simulink library "vmc"  (R2021b)
settings: Solver=VariableStepAuto  StartTime=0.0  StopTime=10.0  RelTol=1e-3
undefined symbols (not defined in the file or in its folder): AVMC_ACCDeltaTqIGain_X_kph, AVMC_ACCDeltaTqIGain_Y_mps2, AVMC_ACCDeltaTqPGain_X_kph, AVMC_ACCDeltaTqPGain_Y_kph, AVMC_ACCLongSteadyCtrl_X_kph, AVMC_AggressJerkPCT4AT_X_kph, AVMC_AggressJerkPCT_X_kph, AVMC_AggressLimitPCT4AT_X_kph, AVMC_AggressLimitPCT_X_kph, AVMC_CCLongSteadyCtrl_X_kph, AVMC_DISCDeltaTqIGain_X_kph, AVMC_DISCDeltaTqIGain_Y_mps2, AVMC_DISCDeltaTqPGain_X_kph, AVMC_DISCDeltaTqPGain_Y_kph, AVMC_DISCTrunAccJerk_X_s, AVMC_DISCTrunAccLimit_X_s, AVMC_ESCRegenOut_X_kph, AVMC_ESCRegenOut_Y_Deg, AVMC_ESCRegenOutEnSpd_X_Deg, AVMC_ISOAccLimit_X_mps, AVMC_ISODecLimit_X_mps, AVMC_ISOJerk_X_mps, AVMC_LatESCRegenOut_X_kph, AVMC_LatESCRegenOut_Y_Deg, AVMC_LongAccDeadZone_X_kph, AVMC_LongAccFiltTsforP2_X_Gps, AVMC_MCPresBaseTq_X_bar, AVMC_MSALongSteadyCtrl_X_kph, AVMC_MSAPedalOvrd2_X_kph, AVMC_MSAPedalOvrd_X_kph, AVMC_MSASpdBand_X_kph, AVMC_MSATqDownEndTq_X_kph, AVMC_MSATqDownTime_X_kph, AVMC_OPDDisSlideRate_X_Deg, AVMC_RDCDetectTime_X_kph, AVMC_RDCDetectTime_Y_pct, AVMC_RDCEnSlideRate_X_Deg, AVMC_RearWhlTqRatio_X_Nm, AVMC_RearWhlTqRatio_Y_gps, AVMC_RearWhlTqSlipGain_X_rat, AVMC_RearWhlTqSlipGain_Y_kph, AVMC_RearWhlTqSTRGGain_X_deg, AVMC_RearWhlTqSTRGGain_Y_kph, AVMC_RWSRrTSA2RWSPos_X_deg, AVMC_RWSSAS2FrtTSA_X_deg, AVMC_RWSVehSPD2RWSCoef_X_kph, AVMC_SoftJerkPCT_X_kph, AVMC_SoftLimitPCT_X_kph, AVMC_StESCYaw_X_kph, AVMC_StESCYaw_Y_Deg, AVMC_StESCYawCom_X_kph, AVMC_StESCYawCom_Y_Gps, AVMC_TMSpdBaseTq_X_rpm, AVMC_VehHoldBDecMap_X_kph, AVMC_VehHoldDecCtrlTime_X_kph, AVMC_VehHoldMCPPass_X_deg, C_TASK_10MS_S, C_TASK_5MS_S, DEG2RAD, ENUM_ACCAVAIL_AVAILABLE ... (+409)
libraries: hcu_lib x74, simulink x68, simulink_extras x3, $bdroot x2
(part 6 of 15)

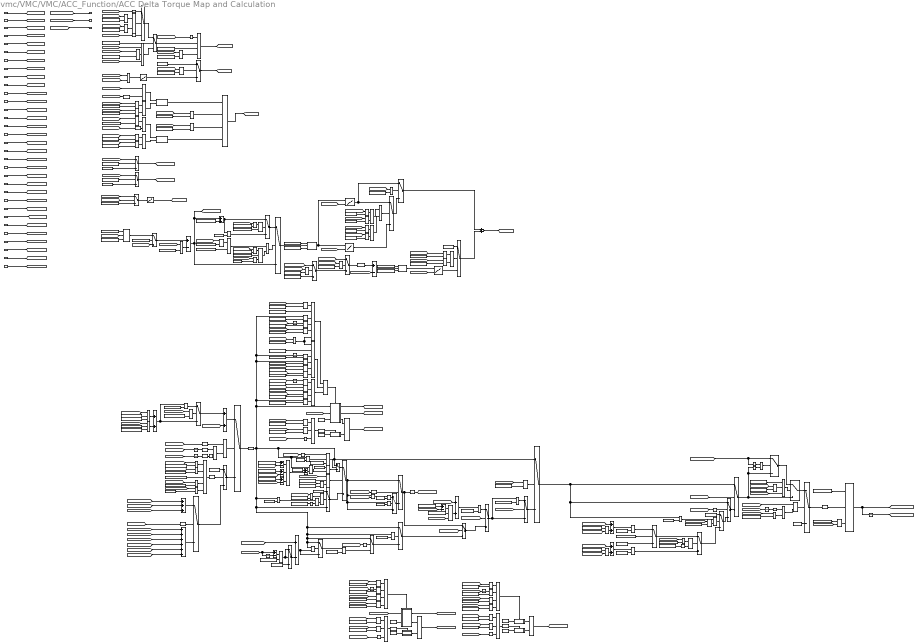
== system vmc/VMC/VMC/ACC_Function/ACC Delta Torque Map and Calculation ==
  note: Deceleration REGEN Torque Control
  note: Deceleration REGEN Torque Control Judgement
  note: Deceleration Torque Control
  note: Deceleration Positive Torque Control
  VVMC_LongAcc_Gps : Inport
  VVMC_ActACCRequiredAccel_mps2 : Inport  Port=2
  VINP_VehSpeed_kph : Inport  Port=3
  VTQD_DriverWhlTqDem_Nm : Inport  Port=4
  VVMC_ADASActive_flg : Inport  Port=5
  VTQD_CoordWhlTqDemFr_Nm : Inport  Port=6
  VTQD_CoordWhlTqDemRr_Nm : Inport  Port=7
  VVMC_ACCPedalOvrd_flg : Inport  Port=8
  VVMC_FeatSetSpdForCalcu_kph : Inport  Port=9
  VVMC_FeatArbitrFinal_enum : Inport  Port=10
  VINP_FrTMSpd_rpm : Inport  Port=11
  VINP_RrTMSpd_rpm : Inport  Port=12
  VINP_MCPressure_bar : Inport  Port=13
  VINP_ESCADASSta_enum : Inport  Port=14
  VINP_FrRBCActive_flg : Inport  Port=15
  VINP_RrRBCActive_flg : Inport  Port=16
  VVMC_FeatReqSpd_kph : Inport  Port=17
  VVMC_MeterIndSpeedForCalcu_kph : Inport  Port=18
  VTQD_SWCResUpSta_flg : Inport  Port=19
  VINP_FrntAxlTrqReqBrk_Nm : Inport  Port=20
  VINP_RearAxlTrqReqBrk_Nm : Inport  Port=21
  VTQR_RrTMTqReq_Nm : Inport  Port=22
  VVMC_ACCVehHoldReq_flg : Inport  Port=23
  VVMC_EstSlope_Deg : Inport  Port=24
  VINP_TargetType_enum : Inport  Port=25
  VVMC_SafetyCtrl_flg : Inport  Port=26
  VTQR_FrTMTqReq_Nm : Inport  Port=27
  task_time_s : Inport  Port=28
  VVMC_TotalAvailBrkRgnTq_Nm : Inport  Port=29
  VVMC_AccelTurnHold_flg : Inport  Port=30
  VVMC_ADASACCSta_enum : Inport  Port=31
  VVMC_TimeGapJudge_flag : Inport  Port=32
  AND{,1,4,10..11,13,15,17..18,20,24,29,31} (13 alike) : Logic  AllPortsSameDT=off  OutDataTypeStr=boolean
  AND12 : Logic  Inputs=3  AllPortsSameDT=off  OutDataTypeStr=boolean
  AND14 : Logic  Operator=OR  AllPortsSameDT=off  OutDataTypeStr=boolean
  AND19 : Logic  Operator=OR  AllPortsSameDT=off  OutDataTypeStr=boolean
  AND2 : Logic  Inputs=4  AllPortsSameDT=off  OutDataTypeStr=boolean
  AND25 : Logic  Inputs=3  AllPortsSameDT=off  OutDataTypeStr=boolean
  AND3 : Logic  Inputs=4  AllPortsSameDT=off  OutDataTypeStr=boolean
  AND30 : Logic  Operator=OR  AllPortsSameDT=off  OutDataTypeStr=boolean
  AND32 : Logic  Inputs=5  AllPortsSameDT=off  OutDataTypeStr=boolean
  AND8 : Logic  Inputs=3  AllPortsSameDT=off  OutDataTypeStr=boolean
  Abs : Abs
  Abs1 : Abs
  Add{,3..4,7..8,10..12,14} (9 alike) : Sum  Inputs=+-
  Add1 : Sum  Inputs=++++++
  Add{5..6,13,15,18,20..21} (7 alike) : Sum
  Add9 : Sum  Inputs=+++
  Cast To Single2 : DataTypeConversion  OutDataTypeStr=single
  Cast To Single3 : DataTypeConversion  OutDataTypeStr=single
  Constant : Constant  Value=TRUE
  Constant1 : Constant  Value=KVMC_ADASNegReqSourceSW_flg
  Constant10 : Constant  Value=KVMC_ADASWhlTqUpperLim_Nm
  Constant100 : Constant  Value=KVMC_ZeroRgnTqSpdCtrlTime_s
  Constant{4,19,22,25,27,29,40,43,45,50..53,58,63..64,66..67,69..70,72..75,81..82,87,89..90,92..93,96,98..99,101,112,114,116..117,119,124..125,129,131..132,149,151,156,163,165,168,170,174} (53 alike) : Constant  Value=ZERO_FLOAT
  Constant11 : Constant  Value=KVMC_ADASWhlTqLowerLim_Nm
  Constant110 : Constant  Value=KVMC_NegReqEnSpd_kph
  Constant113 : Constant  Value=KVMC_ACCLowSpdPosTq_flg
  Constant115 : Constant  Value=KVMC_ACCLowSpdPosTq_flg
  Constant118 : Constant  Value=KVMC_VehHoldTMBaseTqOff_flg
  Constant12 : Constant  Value=KVMC_AccDevLowLim_mps2
  Constant123 : Constant  Value=ENUM_FEATARBITRSTA_DISC
  Constant126 : Constant  Value=KVMC_ReqAccelDeviaEnDec_mps2
  Constant127 : Constant  Value=KVMC_ReqAccelDevia4Tq_flg
  Constant128 : Constant  Value=KVMC_ReqAccelDeviation_mps2
  Constant13 : Constant  Value=KVMC_AccDevUpLim_mps2
  Constant130 : Constant  Value=KVMC_ReqAccelDeviaMinMCP_bar
  Constant138 : Constant  Value=KVMC_ReqAccelLimitSW_flg
  Constant139 : Constant  Value=KVMC_MaxReqAccel_mps2
  Constant14 : Constant  Value=KVMC_ACCSpdDevUpLim_kph
  Constant140 : Constant  Value=KVMC_MinReqAccel_mps2
  Constant146 : Constant  Value=KVMC_ReqAccelDeviaMinMCPSW_flg
  Constant147 : Constant  Value=KVMC_ReqAccelDeviaMinSpd_kph
  Constant148 : Constant  Value=KVMC_ReqAccelDeviaMinSpdSW_flg
  Constant15 : Constant  Value=KVMC_ACCSpdDevLowLim_kph
  Constant157 : Constant  Value=KVMC_AccelTurnHoldZeroTq_flg
  Constant16 : Constant  Value=ENUM_FEATARBITRSTA_ACC
  Constant162 : Constant  Value=KVMC_HoldTqRamp2ZeroSlope_Nmps
  Constant164 : Constant  Value=KVMC_UpHillHoldTqCtrl_flg
  Constant166 : Constant  Value=ENUM_ESCADASSTA_VEHASTANDSTILL
  Constant167 : Constant  Value=KVMC_StandstillTqRamp2ZeroSlope_Nmps
  Constant169 : Constant  Value=KVMC_StandstillTqRampSW_flg
  Constant17 : Constant  Value=ENUM_ADASACCSTA_ACTIVE
  Constant171 : Constant  Value=KVMC_BigDeltaDecGapBand_mps2
  Constant172 : Constant  Value=KVMC_BigDeltaDecJudgeEnBand_mps2
  Constant173 : Constant  Value=KVMC_BigDeltaDecEnGradeBand_deg
  Constant18 : Constant  Value=KVMC_TimeGapTq2Zero_flg
  Constant{2,7..8,20} (4 alike) : Constant  Value=KVMC_HillUpResetTMSpd_rpm
  Constant21 : Constant  Value=ENUM_FEATARBITRSTA_DISC
  Constant23 : Constant  Value=KVMC_ADASNegReqSW_flg
  Constant24 : Constant  Value=KVMC_ACCReqCMdBond_mps2
  Constant26 : Constant  Value=KVMC_AddBRegen2ACCLoop_flg
  Constant3 : Constant  Value=ENUM_ESCADASSTA_VEHASTANDSTILL
  Constant30 : Constant  Value=KVMC_TqSafetyCtrl_flg
  Constant31 : Constant  Value=KVMC_ACCResUpEnAccCMD_mps2
  Constant{6,36..37,62,77,80,88,97} (8 alike) : Constant  Value=KVMC_CutOffNegTqSpd_kph
  Constant38 : Constant  Value=KTQR_FrTMGearEff_c
  Constant39 : Constant  Value=FALSE
  Constant{41,47..48,78..79,91} (6 alike) : Constant  Value=KVMC_ZeroRgnTqSpd_kph
  Constant42 : Constant  Value=KTQD_FrTMTotalGearRatio_gain
  Constant46 : Constant  Value=KVMC_ACCLowSpdTqCtrlSW_flg
  Constant5 : Constant  Value=KVMC_AddBRegen2ACCLoop_flg
  Constant54 : Constant  Value=KVMC_NegReqSwEnSpd_kph
  Constant55 : Constant  Value=KVMC_NegReqSwEnSlope_Deg
  Constant56 : Constant  Value=KVMC_ACCResUpEnGrade_Deg
  Constant57 : Constant  Value=ENUM_TARGETTYPE_NONE
  Constant59 : Constant  Value=KVMC_TqMCPRelFactor_Nm
  Constant60 : Constant  Value=ENUM_FEATARBITRSTA_ACC
  Constant61 : Constant  Value=ENUM_FEATARBITRSTA_ACC
  Constant68 : Constant  Value=KVMC_GradeTqCtrl_flg
  Constant71 : Constant  Value=KVMC_BigDeltaDecGapZeroTq_flg
  Constant76 : Constant  Value=KVMC_DownGradeTqCtrl_flg
  Constant83 : Constant  Value=TRUE
  Constant84 : Constant  Value=KTQD_RrTMTotalGearRatio_gain
  Constant85 : Constant  Value=KTQR_RrTMGearEff_c
  Constant86 : Constant  Value=FALSE
  Constant9 : Constant  Value=KVMC_GravityValue_mps2
  Constant94 : Constant  Value=TRUE
  Constant95 : Constant  Value=FALSE
  Data Type Conversion1 : DataTypeConversion  OutDataTypeStr=single
  Detect Change : simulink/Logic and Bit Operations/Detect Change  vinit=0  OutDataTypeStr=boolean
  Detect Decrease2 : simulink/Logic and Bit Operations/Detect Decrease  vinit=0.0  OutDataTypeStr=boolean
  Detect Decrease3 : simulink/Logic and Bit Operations/Detect Decrease  vinit=0.0  OutDataTypeStr=boolean
  Detect Increase{,1..6,8} (8 alike) : simulink/Logic and Bit Operations/Detect Increase  vinit=0.0  OutDataTypeStr=boolean
  Divide : Product  Inputs=*/*
  Divide1 : Product  Inputs=***
  Divide2 : Product  Inputs=**
  Divide3 : Product  Inputs=*/*
  Divide5 : Product  Inputs=***
  Divide6 : Product  Inputs=**
  Divide7 : Product  Inputs=**
  Equal : RelationalOperator  Operator===  OutDataTypeStr=boolean  RndMeth=Simplest
  Equal1 : RelationalOperator  Operator=<=  OutDataTypeStr=boolean  RndMeth=Simplest
  Equal10 : RelationalOperator  Operator===  OutDataTypeStr=boolean  RndMeth=Simplest
  Equal11 : RelationalOperator  Operator=<  OutDataTypeStr=boolean  RndMeth=Simplest
  Equal12 : RelationalOperator  Operator=>  OutDataTypeStr=boolean  RndMeth=Simplest
  Equal2 : RelationalOperator  Operator=~=  OutDataTypeStr=boolean  RndMeth=Simplest
  Equal3 : RelationalOperator  OutDataTypeStr=boolean  RndMeth=Simplest
  Equal5 : RelationalOperator  OutDataTypeStr=boolean  RndMeth=Simplest
  Equal6 : RelationalOperator  Operator=<  OutDataTypeStr=boolean  RndMeth=Simplest
  Equal7 : RelationalOperator  Operator=>  OutDataTypeStr=boolean  RndMeth=Simplest
  Equal8 : RelationalOperator  Operator=<  OutDataTypeStr=boolean  RndMeth=Simplest
  Equal9 : RelationalOperator  Operator=>  OutDataTypeStr=boolean  RndMeth=Simplest
  InitialCondition: 1 : UnitDelay  SampleTime=-1  HasFrameUpgradeWarning=on
  Logical Operator : Logic  Inputs=4  AllPortsSameDT=off  OutDataTypeStr=boolean
  Logical Operator1 : Logic  Operator=OR  AllPortsSameDT=off  OutDataTypeStr=boolean
  Logical Operator2 : Logic  Inputs=6  AllPortsSameDT=off  OutDataTypeStr=boolean
  Logical Operator3 : Logic  Operator=OR  Inputs=3  AllPortsSameDT=off  OutDataTypeStr=boolean
  Logical Operator4 : Logic  Inputs=6  AllPortsSameDT=off  OutDataTypeStr=boolean
  Logical Operator5 : Logic  Inputs=3  AllPortsSameDT=off  OutDataTypeStr=boolean
  Logical Operator6 : Logic  Inputs=4  AllPortsSameDT=off  OutDataTypeStr=boolean
  Logical Operator7 : Logic  Operator=OR  Inputs=3  AllPortsSameDT=off  OutDataTypeStr=boolean
  Logical Operator8 : Logic  Inputs=4  AllPortsSameDT=off  OutDataTypeStr=boolean
  Logical Operator9 : Logic  Operator=OR  Inputs=3  AllPortsSameDT=off  OutDataTypeStr=boolean
  MVMC_ACCDeltaTqIGain_Z_Nm : Lookup_n-D  BreakpointsForDimension1=AVMC_ACCDeltaTqIGain_Y_mps2  BreakpointsForDimension2=AVMC_ACCDeltaTqIGain_X_kph  Table=MVMC_ACCDeltaTqIGain_Z_Nm  InternalRulePriority=Speed  RndMeth=Simplest  InputSameDT=on
      settings: InputPortMap=u0,u1
  MVMC_ACCDeltaTqPGain_Z_Nm1 : Lookup_n-D  BreakpointsForDimension1=AVMC_ACCDeltaTqPGain_Y_kph  BreakpointsForDimension2=AVMC_ACCDeltaTqPGain_X_kph  Table=MVMC_ACCDeltaTqPGain_Z_Nm  InternalRulePriority=Speed  RndMeth=Simplest  InputSameDT=on
      settings: InputPortMap=u0,u1
  MVMC_DISCDeltaTqIGain_Z_Nm : Lookup_n-D  BreakpointsForDimension1=AVMC_DISCDeltaTqIGain_Y_mps2  BreakpointsForDimension2=AVMC_DISCDeltaTqIGain_X_kph  Table=MVMC_DISCDeltaTqIGain_Z_Nm  InternalRulePriority=Speed  RndMeth=Simplest  InputSameDT=on
      settings: InputPortMap=u0,u1
  MVMC_MCPresBaseTq_Y_Nm : Lookup_n-D  NumberOfTableDimensions=1  BreakpointsForDimension1=AVMC_MCPresBaseTq_X_bar  Table=MVMC_MCPresBaseTq_Y_Nm  InternalRulePriority=Speed  RndMeth=Simplest  InputSameDT=on
  MVMC_TMSpdBaseTq_Y_Nm : Lookup_n-D  NumberOfTableDimensions=1  BreakpointsForDimension1=AVMC_TMSpdBaseTq_X_rpm  Table=MVMC_TMSpdBaseTq_Y_Nm  InternalRulePriority=Speed  RndMeth=Simplest  InputSameDT=on
  Max{,1,4,6..8} (6 alike) : MinMax  Function=max  Inputs=2
  Max2 : MinMax  Inputs=2
  Max3 : MinMax  Inputs=2
  Merge : Merge
  Merge1 : Merge
  Merge2 : Merge
  Min{,1,3..4} (4 alike) : MinMax  Inputs=2
  Min2 : MinMax  Function=max  Inputs=2
  NOT{,1..5,7,9,12..13,20} (11 alike) : Logic  Operator=NOT  AllPortsSameDT=off  OutDataTypeStr=boolean
  OR{,1,6,11,18} (5 alike) : Logic  Operator=OR  AllPortsSameDT=off  OutDataTypeStr=boolean
  OR2 : Logic  Operator=OR  Inputs=3  AllPortsSameDT=off  OutDataTypeStr=boolean
  OR3 : Logic  Operator=OR  Inputs=3  AllPortsSameDT=off  OutDataTypeStr=boolean
  OR5 : Logic  AllPortsSameDT=off  OutDataTypeStr=boolean
  Product1 : Product
  Relational Operator{,2..4,7,16,32..33,38,44,47} (11 alike) : RelationalOperator  Operator=>  OutDataTypeStr=boolean  RndMeth=Simplest
  Relational Operator{1,9,11,14..15,21..23,26,28,30..31,35,41,45,49..50,57,67} (19 alike) : RelationalOperator  Operator=<  OutDataTypeStr=boolean  RndMeth=Simplest
  Relational Operator{8,10,12,24..25,29,36..37,39,42..43} (11 alike) : RelationalOperator  OutDataTypeStr=boolean  RndMeth=Simplest
  Relational Operator{5..6,17,19,55,73} (6 alike) : RelationalOperator  Operator===  OutDataTypeStr=boolean  RndMeth=Simplest
  Relational Operator{18,20,27,34,40,56,66,71,74} (9 alike) : RelationalOperator  Operator=<=  OutDataTypeStr=boolean  RndMeth=Simplest
  Relay : Relay  OnSwitchValue=KVMC_ACCTq2ZeroEnMCPress2_bar  OffSwitchValue=KVMC_ACCTq2ZeroDisMCPress2_bar  OutDataTypeStr=boolean
  Relay1 : Relay  OnSwitchValue=KVMC_ACCTq2ZeroEnMCPress_bar  OffSwitchValue=KVMC_ACCTq2ZeroDisMCPress_bar  OutDataTypeStr=boolean
  SR_Latch : hcu_lib/Basic_Blocks/SR_Latch
  SR_Latch1 : hcu_lib/Basic_Blocks/SR_Latch
  Saturation Dynamic{1,3..5} (4 alike) : simulink/Discontinuities/Saturation Dynamic  OutMin=[]  OutMax=[]  OutDataTypeStr=Inherit: Same as second input  OutDataType=fixdt(1, 16)  OutScaling=2^-10  DoSatur=off
  Switch{,1..19,21..24,27,29,33..35,37..39,41..43} (35 alike) : Switch  Criteria=u2 > Threshold
  Triggered Subsystem : Subsystem  TreatAsAtomicUnit=on
  Triggered Subsystem1 : Subsystem  TreatAsAtomicUnit=on
  Triggered Subsystem2 : Subsystem  TreatAsAtomicUnit=on
  Triggered Subsystem3 : Subsystem  TreatAsAtomicUnit=on
  Triggered Subsystem4 : Subsystem  TreatAsAtomicUnit=on
  Triggered Subsystem5 : Subsystem  TreatAsAtomicUnit=on
  Unit Delay{,1..9} (10 alike) : UnitDelay  SampleTime=-1  HasFrameUpgradeWarning=on
  u2 > 0 : Switch  Criteria=u2 > Threshold
  u2 > 0 (1) : Switch  Criteria=u2 > Threshold
  u2 > 0 (3) : Switch  Criteria=u2 > Threshold
  u2 > 0 (4) : Switch  Criteria=u2 > Threshold
  VVMC_ADASWhlTqCal_Nm : Outport
  VVMC_ADASNegReq_flg : Outport  Port=2
  VVMC_ACCLowSpdTqCtrl_flg : Outport  Port=3
  wires:
  VVMC_FeatReqSpd_kph/1 -> [VVMC_FeatReqSpd_kph]
  [VINP_RrTMSpd_rpm] -> Relational Operator2/1
  [VVMC_ACCVehHoldReq_flg] -> AND4/1
  MVMC_MCPresBaseTq_Y_Nm/1 -> [VVMC_MCPresBaseTq_Nm]  "VVMC_MCPresBaseTq_Nm"
  Switch1/1 -> MVMC_MCPresBaseTq_Y_Nm/1
  [VINP_MCPressure_bar] -> Switch1/1
  Relational Operator/1 -> OR/1
  Equal/1 -> AND1/1
  OR/1 -> SR_Latch/2
  [VINP_FrTMSpd_rpm] -> Relational Operator/1
  [VINP_ESCADASSta_enum] -> Equal/1
  [VINP_RrTMSpd_rpm] -> Relational Operator4/1
  AND1/1 -> SR_Latch1/1
  Relational Operator2/1 -> OR/2
  OR1/1 -> SR_Latch1/2
  Constant19/1 -> Switch1/3
  Constant8/1 -> Relational Operator3/2
  Relational Operator4/1 -> OR1/2
  [VVMC_MCPreBaseTqEn_flg] -> Switch1/2
  [VINP_FrTMSpd_rpm] -> Relational Operator3/1
  Constant7/1 -> Relational Operator4/2
  Constant2/1 -> Relational Operator2/2
  Detect Increase3/1 -> AND1/2
  SR_Latch/1 -> AND3/1  "VVMC_HillUpHoldReqEn_flg"
  AND3/1 -> [VVMC_MCPreBaseTqEn_flg]  "VVMC_MCPreBaseTqEn_flg"
  SR_Latch1/1 -> AND3/4  "VVMC_HillUpESCStaEn_flg"
  Constant3/1 -> Equal/2
  Constant20/1 -> Relational Operator/2
  Relational Operator3/1 -> OR1/1
  VINP_FrTMSpd_rpm/1 -> [VINP_FrTMSpd_rpm]
  VINP_RrTMSpd_rpm/1 -> [VINP_RrTMSpd_rpm]
  VINP_MCPressure_bar/1 -> [VINP_MCPressure_bar]
  VINP_ESCADASSta_enum/1 -> [VINP_ESCADASSta_enum]
  VINP_FrRBCActive_flg/1 -> [VINP_FrRBCActive_flg]
  VINP_RrRBCActive_flg/1 -> [VINP_RrRBCActive_flg]
  VVMC_FeatArbitrFinal_enum/1 -> [VVMC_FeatArbitrFinal_enum]
  VVMC_LongAcc_Gps/1 -> [VVMC_LongAcc_Gps]
  VVMC_ActACCRequiredAccel_mps2/1 -> [VVMC_ActACCRequiredAccel_mps2]
  VINP_VehSpeed_kph/1 -> [VINP_VehSpeed_kph]
  VTQD_DriverWhlTqDem_Nm/1 -> [VTQD_DriverWhlTqDem_Nm]
  VVMC_ADASActive_flg/1 -> [VVMC_ADASActive_flg]
  [VVMC_ADASWhlTqCal_Nm] -> VVMC_ADASWhlTqCal_Nm/1
  VTQD_CoordWhlTqDemFr_Nm/1 -> [VTQD_CoordWhlTqDemFr_Nm]
  VTQD_CoordWhlTqDemRr_Nm/1 -> [VTQD_CoordWhlTqDemRr_Nm]
  VVMC_ACCPedalOvrd_flg/1 -> [VVMC_ACCPedalOvrd_flg]
  VVMC_FeatSetSpdForCalcu_kph/1 -> [VVMC_FeatSetSpdForCalcu_kph]
  VINP_RearAxlTrqReqBrk_Nm/1 -> [VINP_RearAxlTrqReqBrk_Nm]
  VINP_FrntAxlTrqReqBrk_Nm/1 -> [VINP_FrntAxlTrqReqBrk_Nm]
  VTQD_SWCResUpSta_flg/1 -> [VTQD_SWCResUpSta_flg]
  VVMC_MeterIndSpeedForCalcu_kph/1 -> [VVMC_MeterIndSpeedForCalcu_kph]
  [VTQD_SWCResUpSta_flg] -> Detect Increase2/1
  AND4/1 -> SR_Latch/1
  [VVMC_ActACCRequiredAccel_mps2] -> Relational Operator7/1
  Constant31/1 -> Relational Operator7/2
  [VTQD_SWCResUpSta_flg] -> Detect Increase3/1
  [VINP_FrntAxlTrqReqBrk_Nm] -> Switch3/1
  [VINP_RearAxlTrqReqBrk_Nm] -> Switch4/1
  Constant25/1 -> Switch3/3
  Constant27/1 -> Switch4/3
  Constant26/1 -> Switch4/2
  Switch4/1 -> [VVMC_RearAxlTrqReqBrk_Nm]  "VVMC_RearAxlTrqReqBrk_Nm"
  Switch3/1 -> [VVMC_FrntAxlTrqReqBrk_Nm]  "VVMC_FrntAxlTrqReqBrk_Nm"
  Constant5/1 -> Switch3/2
  [VVMC_ADASNegReq_flg] -> VVMC_ADASNegReq_flg/1
  VTQR_RrTMTqReq_Nm/1 -> [VTQR_RrTMTqReq_Nm]
  VVMC_ACCVehHoldReq_flg/1 -> [VVMC_ACCVehHoldReq_flg]
  [VVMC_EstSlope_Deg] -> Relational Operator16/1
  Relational Operator16/1 -> AND3/3
  Constant56/1 -> Relational Operator16/2
  VVMC_EstSlope_Deg/1 -> [VVMC_EstSlope_Deg]
  VINP_TargetType_enum/1 -> [VINP_TargetType_enum]
  VVMC_SafetyCtrl_flg/1 -> [VVMC_SafetyCtrl_flg]
  VTQR_FrTMTqReq_Nm/1 -> [VTQR_FrTMTqReq_Nm]
  [VVMC_ACCLowSpdTqCtrl_flg] -> VVMC_ACCLowSpdTqCtrl_flg/1
  task_time_s/1 -> [task_time_s]
  MVMC_TMSpdBaseTq_Y_Nm/1 -> Switch/3
  [VVMC_ActACCRequiredAccel_mps2] -> Relational Operator1/1
  AND15/1 -> Switch/2
  Relay/1 -> Switch13/1
  Constant24/1 -> Relational Operator1/2
  [VVMC_ACCVehHoldReq_flg] -> AND15/1
  Switch2/1 -> AND2/2  "VVMC_ADASNegReqAct_flg"
  AND2/1 -> [VVMC_ADASNegReq_flg]  "VVMC_ADASNegReq_flg"
  [VINP_FrRBCActive_flg] -> OR2/1
  Constant23/1 -> AND2/3
  Constant1/1 -> Switch2/2
  [VINP_RrTMSpd_rpm] -> Min/2
  [VVMC_MCPreBaseTqEn_flg] -> NOT2/1
  Equal5/1 -> AND2/4
  [VINP_VehSpeed_kph] -> Equal5/1
  [VINP_FrTMSpd_rpm] -> Min/1
  Switch13/1 -> Switch2/1
  Constant110/1 -> Equal5/2
  [VINP_MCPressure_bar] -> Relay/1
  [VINP_VehSpeed_kph] -> Equal1/1
  Equal3/1 -> AND10/2
  Relay1/1 -> Switch13/3
  Relational Operator1/1 -> OR2/2
  Switch/1 -> [VVMC_TMSpdBaseTq_Nm]  "VVMC_TMSpdBaseTq_Nm"
  Constant54/1 -> Equal1/2
  Constant118/1 -> AND15/2
  [VINP_MCPressure_bar] -> Relay1/1
  AND10/1 -> Switch13/2
  Constant55/1 -> Equal3/2
  [VVMC_EstSlope_Deg] -> Equal3/1
  Equal1/1 -> AND10/1
  Min/1 -> MVMC_TMSpdBaseTq_Y_Nm/1
  NOT2/1 -> AND2/1
  OR2/1 -> Switch2/3
  [VINP_RrRBCActive_flg] -> OR2/3
  Constant119/1 -> Switch/1
  Switch29/1 -> Switch22/3
  [VINP_VehSpeed_kph] -> Relational Operator21/1
  [VINP_VehSpeed_kph] -> Relational Operator20/1
  Relational Operator11/1 -> Logical Operator/2
  Merge2/1 -> [VVMC_ZeroRgnTqSpdCtrl_flg]  "VVMC_ZeroRgnTqSpdCtrl_flg"
  [VVMC_ActACCRequiredAccel_mps2] -> Relational Operator37/1
  Relational Operator50/1 -> Switch29/2
  Constant48/1 -> Add4/1
  Relational Operator73/1 -> OR6/2
  Constant86/1 -> Triggered Subsystem3/1(In1)
  Relational Operator31/1 -> Logical Operator4/1
  Relational Operator39/1 -> Logical Operator6/1
  [VVMC_ActACCRequiredAccel_mps2] -> Relational Operator41/1
  NOT12/1 -> AND14/2
  Logical Operator2/1 -> OR3/2
  Constant93/1 -> Relational Operator42/2
  Relational Operator25/1 -> Logical Operator2/3
  Max1/1 -> Switch23/1
  Detect Increase5/1 -> Triggered Subsystem3/Trigger
  Constant115/1 -> NOT12/1
  Unit Delay4/1 -> NOT4/1
  Logical Operator/1 -> OR3/3
  Detect Increase6/1 -> Triggered Subsystem5/Trigger
  [VVMC_LastADASWhlTqCal_Nm] -> Add12/1
  [VINP_VehSpeed_kph] -> Relational Operator8/1
  Switch8/1 -> Switch43/3
  [VVMC_ADASActive_flg] -> NOT1/1
  Constant63/1 -> Min2/2
  Logical Operator3/1 -> Detect Increase/1
  Constant29/1 -> Relational Operator10/2
  Triggered Subsystem2/1(Out1) -> Merge/2
  Relational Operator8/1 -> Logical Operator3/1
  Unit Delay/1 -> Relational Operator12/1
  [VVMC_TMSpdBaseTq_Nm] -> Add1/3
  Logical Operator1/1 -> Switch6/2
  Constant36/1 -> Relational Operator11/2
  NOT1/1 -> Logical Operator3/3
  [VINP_MCPressure_bar] -> Add11/1, Unit Delay5/1
  [VVMC_FrntAxlTrqReqBrk_Nm] -> Add1/5
  [VTQD_CoordWhlTqDemFr_Nm] -> Add9/1
  Divide2/1 -> Switch15/1, Switch15/2
  Constant92/1 -> Relational Operator41/2
  Constant74/1 -> Switch5/3
  Constant84/1 -> Divide5/2
  Relational Operator15/1 -> Logical Operator/4
  Constant11/1 -> Max6/1
  Constant113/1 -> AND8/3
  [VVMC_ActACCRequiredAccel_mps2] -> Relational Operator10/1
  Triggered Subsystem3/1(Out1) -> Merge1/2
  Constant114/1 -> Relational Operator49/2
  AND13/1 -> Switch21/2
  Constant69/1 -> Switch15/3
  [VVMC_LastADASWhlTqCal_Nm] -> Relational Operator39/1
  Add14/1 -> Divide3/1
  Constant101/1 -> Max2/2
  Switch23/1 -> Switch17/3
  Constant70/1 -> Relational Operator26/2
  [VVMC_ADASActive_flg] -> OR5/1
  Abs1/1 -> Relational Operator18/2
  [VVMC_MCPresBaseTq_Nm] -> Add1/4
  [VINP_VehSpeed_kph] -> Relational Operator44/1
  Switch11/1 -> u2 > 0 (3)/3, u2 > 0 (4)/3, Abs1/1
  Constant61/1 -> Relational Operator19/2
  Abs/1 -> Relational Operator18/1
  Relational Operator19/1 -> AND12/2
  Constant87/1 -> Relational Operator37/2
  Constant68/1 -> Logical Operator2/2
  Switch10/1 -> Min2/1
  Constant64/1 -> Relational Operator22/2
  Constant10/1 -> Saturation Dynamic3/1
  Min2/1 -> Switch16/3
  [VTQR_RrTMTqReq_Nm] -> Divide5/1
  Triggered Subsystem1/2(Out2) -> [VVMC_ACCLowSpdCtrlEnSpd_kph]  "VVMC_ACCLowSpdCtrlEnSpd_kph"
  NOT9/1 -> Logical Operator9/3
  Switch6/1 -> Cast To Single2/1
  Logical Operator8/1 -> Triggered Subsystem4/Trigger
  Cast To Single2/1 -> Relational Operator9/1, Switch10/1, Switch16/1, Relational Operator26/1, Switch19/1, Switch21/3, Relational Operator49/1, Switch17/1, Switch27/1, Max4/1, Relational Operator47/1, Relational Operator30/1, Unit Delay3/1, Relational Operator23/1, Relational Operator15/1, Triggered Subsystem1/1(In1)  "VVMC_OriADASWhlTq_Nm"
  Add11/1 -> Divide2/1
  Unit Delay7/1 -> [VVMC_LastACCLowSpdTq_Nm]
  Detect Increase1/1 -> Logical Operator1/1
  [VVMC_ZeroRgnTqSpdCtrl_flg] -> Switch24/2
  Triggered Subsystem/1(Out1) -> Merge1/1
  Add15/1 -> Max2/1
  Constant46/1 -> Logical Operator5/2
  Add5/1 -> Switch6/1
  Relational Operator34/1 -> Logical Operator6/4
  Divide1/1 -> Add13/1
  Triggered Subsystem4/1(Out1) -> [VVMC_ZeroRgnTqSpdCtrlTq_Nm]  "VVMC_ZeroRgnTqSpdCtrlTq_Nm"
  Unit Delay9/1 -> Relational Operator42/1
  Detect Decrease2/1 -> Switch8/2
  Add13/1 -> Switch9/3, Min3/1
  [VVMC_SafetyCtrl_flg] -> AND12/3
  [VVMC_LastADASWhlTqCal_Nm] -> Relational Operator45/1
  Relational Operator32/1 -> Logical Operator4/6, Logical Operator2/1
  [VVMC_LastADASWhlTqCal_Nm] -> Triggered Subsystem4/1(In1)
  Constant96/1 -> Relational Operator43/2
  [VINP_VehSpeed_kph] -> Relational Operator40/1
  Constant94/1 -> Triggered Subsystem4/2(In2)
  Divide/1 -> Add/2
  Constant67/1 -> Relational Operator25/2
  Constant90/1 -> Relational Operator39/2
  Relational Operator44/1 -> Logical Operator9/1
  Relational Operator30/1 -> Logical Operator4/3
  Switch21/1 -> Switch12/3
  [VVMC_ActACCRequiredAccel_mps2] -> Unit Delay6/1
  [VVMC_ActACCRequiredAccel_mps2] -> Relational Operator43/1
  Constant97/1 -> Relational Operator44/2
  [VVMC_ADASActive_flg] -> NOT9/1
  Add/1 -> Max4/2
  Relational Operator29/1 -> Logical Operator4/4
  Relational Operator45/1 -> Logical Operator8/1
  Constant80/1 -> Relational Operator34/2
  Constant81/1 -> Relational Operator35/2
  Triggered Subsystem5/1(Out1) -> Merge2/2
  Constant98/1 -> Relational Operator45/2
  Constant95/1 -> Triggered Subsystem5/1(In1)
  Constant6/1 -> Relational Operator8/2
  [VVMC_ActACCRequiredAccel_mps2] -> Unit Delay9/1
  Switch18/1 -> Switch24/3
  Add1/1 -> Switch8/3
  Constant100/1 -> Divide3/2
  Triggered Subsystem4/2(Out2) -> Merge2/1
  Constant89/1 -> Max1/2
  Switch7/1 -> Switch11/3
  [VVMC_FeatArbitrFinal_enum] -> Relational Operator19/1
  [VVMC_RgnProhibited_flg] -> Switch23/2
  [VINP_VehSpeed_kph] -> Relational Operator31/1
  [task_time_s] -> Divide3/3
  Merge1/1 -> [VVMC_RgnProhibited_flg]  "VVMC_RgnProhibited_flg"
  Constant53/1 -> Switch21/1
  Relational Operator38/1 -> Logical Operator7/1
  [VVMC_LastADASWhlTqCal_Nm] -> Abs/1, u2 > 0 (4)/1
  Constant88/1 -> Relational Operator38/2
  Triggered Subsystem1/3(Out3) -> Merge/1
  [VVMC_ADASActive_flg] -> NOT7/1
  Relational Operator36/1 -> Logical Operator6/2
  Logical Operator6/1 -> Triggered Subsystem/Trigger
  Max2/1 -> Switch24/1
  Constant82/1 -> Relational Operator36/2
  Constant99/1 -> Add14/1
  [VINP_VehSpeed_kph] -> Relational Operator34/1
  Unit Delay8/1 -> Relational Operator36/1
  Relational Operator35/1 -> Logical Operator6/3
  NOT7/1 -> Logical Operator7/3
  Relational Operator12/1 -> Logical Operator/1
  [VVMC_LastACCLowSpdTq_Nm] -> Max/2
  Switch12/1 -> Switch29/3, Relational Operator50/1, Max/1, Switch22/1
  Switch15/1 -> Add12/2
  Constant117/1 -> Max3/2
  Add9/1 -> Switch8/1
  [VVMC_ActACCRequiredAccel_mps2] -> Relational Operator24/1
  [VVMC_ACCLowSpdCtrlEnSpd_kph] -> Add4/2
  [VVMC_ActACCRequiredAccel_mps2] -> Relational Operator35/1
  Min1/1 -> Switch27/3
  Detect Increase/1 -> Triggered Subsystem2/Trigger
  Relational Operator20/1 -> AND13/1
  Relational Operator47/1 -> AND8/2
  Max/1 -> Max3/1
  Relational Operator43/1 -> Logical Operator9/2
  Constant47/1 -> Add3/1
  Logical Operator9/1 -> Detect Increase6/1
  [VVMC_ACCLowSpdTqCtrl_flg] -> Detect Increase4/1
  Constant4/1 -> Relational Operator24/2
  Unit Delay5/1 -> Add11/2
  Max3/1 -> Switch29/1
  Detect Increase4/1 -> Switch22/2
  Constant78/1 -> Relational Operator32/2
  Constant79/1 -> Relational Operator33/2
  [VINP_VehSpeed_kph] -> Relational Operator32/1
  [VVMC_ACCLowSpdCtrlEnSpd_kph] -> Relational Operator33/1
  Constant76/1 -> Logical Operator4/2
  [VVMC_ZeroRgnTqSpdCtrlTq_Nm] -> Add14/2
  Constant77/1 -> Relational Operator31/2
  Constant75/1 -> Relational Operator30/2
  Logical Operator4/1 -> OR3/1
  Constant73/1 -> Relational Operator29/2
  Relational Operator42/1 -> Logical Operator8/2
  Constant72/1 -> Relational Operator28/2
  [VVMC_ADASActive_flg] -> Detect Increase1/1
  Relational Operator28/1 -> Logical Operator4/5
  AND12/1 -> u2 > 0 (3)/2
  [VVMC_ActACCRequiredAccel_mps2] -> Relational Operator28/1
  [VVMC_RearAxlTrqReqBrk_Nm] -> Add1/6
  Constant40/1 -> Relational Operator14/2
  Relational Operator41/1 -> Logical Operator8/3
  Constant83/1 -> Triggered Subsystem/1(In1)
  Switch24/1 -> Switch23/3, Max1/1
  OR6/1 -> OR5/2
  [VINP_VehSpeed_kph] -> Unit Delay/1
  [VINP_VehSpeed_kph] -> Triggered Subsystem1/2(In2)
  Unit Delay3/1 -> Relational Operator25/1
  Relational Operator26/1 -> Switch19/2
  AND14/1 -> AND13/2
  Logical Operator7/1 -> Detect Increase5/1
  OR5/1 -> Switch5/2
  Constant38/1 -> Divide1/3
  Switch22/1 -> Unit Delay7/1, Switch18/1  "VVMC_ACCLowSpdTq_Nm"
  [VVMC_ACCLowSpdTqCtrl_flg] -> Logical Operator5/1
  Saturation Dynamic3/1 -> [VVMC_ADASWhlTqCal_Nm], InitialCondition: 1/1  "VVMC_ADASWhlTqCal_Nm"
  OR3/1 -> Triggered Subsystem1/Trigger
  Relational Operator23/1 -> Logical Operator2/4
  [VVMC_ActACCRequiredAccel_mps2] -> Relational Operator22/1
  [VTQR_FrTMTqReq_Nm] -> Divide1/1
  Switch27/1 -> Switch12/1
  u2 > 0 (4)/1 -> u2 > 0 (3)/1
  Relational Operator21/1 -> Logical Operator2/5
  Constant62/1 -> Relational Operator21/2
  Max6/1 -> Saturation Dynamic3/3
  Relational Operator10/1 -> Logical Operator3/2
  Unit Delay6/1 -> Relational Operator29/1
  Relational Operator18/1 -> u2 > 0 (4)/2
  [VINP_VehSpeed_kph] -> Relational Operator11/1
  Constant/1 -> Triggered Subsystem1/3(In3)
  Add10/1 -> Divide/3
  Constant112/1 -> Relational Operator47/2
  [VVMC_MCPreBaseTqEn_flg] -> Switch11/2
  Logical Operator5/1 -> Switch12/2
  AND/1 -> Logical Operator1/2
  Constant52/1 -> Min1/1
  [VVMC_ACCVehHoldReq_flg] -> NOT3/1
  Relational Operator9/1 -> Switch10/2
  Add12/1 -> Relational Operator9/2, Switch10/3  "VVMC_ACCTqRampOutByMCP_Nm"
  Add4/1 -> Divide/2
  [VVMC_LastADASWhlTqCal_Nm] -> Add15/1
  Add3/1 -> Divide/1
  [VVMC_ADASNegReq_flg] -> Detect Decrease2/1
  Divide5/1 -> Add13/2
  Relational Operator24/1 -> Switch17/2
  Constant85/1 -> Divide5/3
  Constant50/1 -> Add10/1
  Relational Operator37/1 -> Logical Operator7/2
  Constant37/1 -> Relational Operator12/2
  [VVMC_ACCDeltaTq_Nm] -> Add9/3
  Relational Operator22/1 -> Logical Operator2/6
  Constant66/1 -> Relational Operator23/2
  Constant45/1 -> Relational Operator15/2
  Relational Operator40/1 -> Logical Operator8/4
  InitialCondition: 1/1 -> [VVMC_LastADASWhlTqCal_Nm]  "VVMC_LastADASWhlTqCal_Nm"
  Constant42/1 -> Divide1/2
  [VVMC_ActACCRequiredAccel_mps2] -> Relational Operator14/1
  Relational Operator14/1 -> Logical Operator/3
  [VVMC_ACCDeltaTq_Nm] -> Add1/2
  u2 > 0 (3)/1 -> Switch5/1
  [VVMC_LastADASWhlTqCal_Nm] -> Add1/1
  [VVMC_ACCLowSpdTqLimit_Nm] -> Add10/2
  Triggered Subsystem1/1(Out1) -> [VVMC_ACCLowSpdTqLimit_Nm]  "VVMC_ACCLowSpdTqLimit_Nm"
  NOT3/1 -> Switch7/2
  Constant116/1 -> Relational Operator50/2
  Relational Operator33/1 -> Logical Operator5/3
  [VINP_VehSpeed_kph] -> Add3/2
  Constant51/1 -> Add/1
  [VVMC_ACCLowSpdTqCtrl_flg] -> Switch18/2
  [VTQD_CoordWhlTqDemRr_Nm] -> Add9/2
  Merge/1 -> [VVMC_ACCLowSpdTqCtrl_flg]  "VVMC_ACCLowSpdTqCtrl_flg"
  [VVMC_ACCPedalOvrd_flg] -> Unit Delay4/1
  Constant39/1 -> Triggered Subsystem2/1(In1)
  Constant91/1 -> Relational Operator40/2
  Constant41/1 -> Relational Operator20/2
  Divide3/1 -> Add15/2
  [VVMC_ACCDeltaTq_Nm] -> Add5/2
  [VINP_VehSpeed_kph] -> Relational Operator38/1
  Cast To Single3/1 -> Saturation Dynamic3/2
  Constant59/1 -> Divide2/2
  Switch5/1 -> Cast To Single3/1
  Relational Operator49/1 -> AND14/1
  AND8/1 -> Switch27/2
  Constant30/1 -> AND12/1
  [VVMC_ActACCRequiredAccel_mps2] -> Unit Delay8/1
  Switch17/1 -> Relational Operator71/1, Switch7/1, Switch11/1
  NOT13/1 -> AND8/1
  [VVMC_ADASNegReq_flg] -> NOT13/1
  Constant12/1 -> Saturation Dynamic4/3
  Saturation Dynamic4/1 -> MVMC_DISCDeltaTqIGain_Z_Nm/1, MVMC_ACCDeltaTqIGain_Z_Nm/1  "VVMC_ActAccDev_mps2"
  Switch33/1 -> Add6/1  "VVMC_ACCDeltaTqIGain_Nm"
  Saturation Dynamic5/1 -> MVMC_ACCDeltaTqPGain_Z_Nm1/1  "VVMC_ACCActSpdDev_kph"
  [VVMC_LongAcc_Gps] -> Product1/1
  Constant16/1 -> Relational Operator5/2
  [VVMC_FeatArbitrFinal_enum] -> Relational Operator6/1
  [VVMC_FeatArbitrFinal_enum] -> Relational Operator5/1
  [VVMC_FeatReqSpd_kph] -> u2 > 0 (1)/1
  Constant15/1 -> Saturation Dynamic5/3
  Equal2/1 -> AND11/1
  Constant128/1 -> Add18/2
  Product1/1 -> Add7/2
  Constant21/1 -> Relational Operator6/2
  Constant60/1 -> Relational Operator17/2
  u2 > 0/1 -> Data Type Conversion1/1
  u2 > 0 (1)/1 -> u2 > 0/3
  [VVMC_MeterIndSpeedForCalcu_kph] -> Add8/2
  Add7/1 -> [VVMC_ACCDeltaAccel_mps2], Add18/1, Switch35/3
  Switch38/1 -> Switch35/1
  Constant127/1 -> AND18/2
  [VVMC_LongAcc_Gps] -> Equal6/1
  AND17/1 -> AND19/1
  [VVMC_ActACCRequiredAccel_mps2] -> Equal7/1
  [VINP_VehSpeed_kph] -> MVMC_DISCDeltaTqIGain_Z_Nm/2
  Relational Operator56/1 -> AND18/1
  Constant125/1 -> Equal7/2
  [VINP_TargetType_enum] -> Equal2/1
  MVMC_DISCDeltaTqIGain_Z_Nm/1 -> Switch33/1, Switch34/1  "VVMC_DISCDeltaTqIGain_Nm"
  Constant124/1 -> Equal6/2
  Data Type Conversion1/1 -> Add8/1
  Relational Operator5/1 -> u2 > 0/2
  Add6/1 -> [VVMC_ACCDeltaTq_Nm]  "VVMC_ACCDeltaTq_Nm"
  MVMC_ACCDeltaTqIGain_Z_Nm/1 -> Switch34/3  "VVMC_ACCDeltaTqIGain_Nm"
  Add18/1 -> Min4/1, Switch38/1
  Constant13/1 -> Saturation Dynamic4/1
  [VVMC_FeatArbitrFinal_enum] -> Relational Operator55/1
  Relational Operator55/1 -> Switch33/2
  Constant9/1 -> Product1/2
  [VINP_VehSpeed_kph] -> MVMC_ACCDeltaTqIGain_Z_Nm/2
  Equal6/1 -> AND17/1
  Add8/1 -> Saturation Dynamic5/2
  [VINP_VehSpeed_kph] -> MVMC_ACCDeltaTqPGain_Z_Nm1/2
  Constant129/1 -> Min4/2
  Switch35/1 -> Saturation Dynamic4/2
  Constant123/1 -> Relational Operator55/2
  Constant22/1 -> u2 > 0 (1)/3
  Constant14/1 -> Saturation Dynamic5/1
  Equal7/1 -> AND17/2
  AND11/1 -> Switch14/2
  Relational Operator6/1 -> u2 > 0 (1)/2
  [VVMC_FeatSetSpdForCalcu_kph] -> u2 > 0/1
  MVMC_ACCDeltaTqPGain_Z_Nm1/1 -> Switch14/3
  AND18/1 -> OR11/1
  Relational Operator17/1 -> AND11/2
  [VVMC_FeatArbitrFinal_enum] -> Relational Operator17/1
  Constant57/1 -> Equal2/2
  Switch34/1 -> Switch33/3
  Constant58/1 -> Switch14/1
  Switch14/1 -> Add6/2  "VVMC_ACCDeltaTqPGain_Nm"
  AND19/1 -> Switch34/2
  Constant131/1 -> Equal8/2
  [VVMC_ActACCRequiredAccel_mps2] -> Equal8/1
  Equal8/1 -> AND20/1
  AND20/1 -> AND19/2
  Equal9/1 -> AND20/2
  [VVMC_ACCDeltaAccel_mps2] -> Equal9/1
  Constant132/1 -> Equal9/2
  Constant126/1 -> Relational Operator56/2
  [VVMC_ActACCRequiredAccel_mps2] -> Relational Operator56/1
  Max4/1 -> Min1/2
  Switch19/1 -> Switch18/3
  [VINP_MCPressure_bar] -> Relational Operator57/1
  Constant130/1 -> Relational Operator57/2
  Relational Operator57/1 -> AND24/1
  Min4/1 -> Switch38/3
  AND24/1 -> Switch38/2
  Constant146/1 -> AND24/2
  OR11/1 -> Switch35/2
  Constant148/1 -> AND25/2
  Constant147/1 -> Relational Operator66/2
  [VINP_VehSpeed_kph] -> Relational Operator66/1
  Relational Operator66/1 -> AND25/1
  AND25/1 -> OR11/2
  Relational Operator67/1 -> AND25/3
  [VVMC_ActACCRequiredAccel_mps2] -> Relational Operator67/1
  Constant149/1 -> Relational Operator67/2
  NOT4/1 -> OR6/1
  Switch39/1 -> Switch7/3
  Constant151/1 -> Relational Operator71/2
  Relational Operator71/1 -> OR18/1
  Detect Increase2/1 -> AND4/2
  Relational Operator7/1 -> AND3/2
  Constant156/1 -> Switch39/1
  VVMC_TotalAvailBrkRgnTq_Nm/1 -> [VVMC_TotalAvailBrkRgnTq_Nm]
  [VVMC_TotalAvailBrkRgnTq_Nm] -> Max6/2
  VVMC_AccelTurnHold_flg/1 -> [VVMC_AccelTurnHold_flg]
  OR18/1 -> Switch39/2
  [VVMC_AccelTurnHold_flg] -> AND29/1
  AND29/1 -> OR18/2
  Constant157/1 -> AND29/2
  Switch41/1 -> Switch39/3
  [task_time_s] -> Divide6/2
  Constant162/1 -> Divide6/1
  [VVMC_LastADASWhlTqCal_Nm] -> Add20/1
  Divide6/1 -> Add20/2
  Add20/1 -> Max7/1
  Constant163/1 -> Max7/2
  Equal10/1 -> AND30/1
  Constant164/1 -> NOT20/1
  Constant166/1 -> Equal10/2
  [VINP_ESCADASSta_enum] -> Equal10/1
  NOT20/1 -> AND30/2
  AND30/1 -> Switch41/2
  Switch42/1 -> Switch41/1
  Max7/1 -> Switch41/3
  Constant168/1 -> Max8/2
  Add21/1 -> Max8/1
  Divide7/1 -> Add21/2
  [VVMC_LastADASWhlTqCal_Nm] -> Add21/1
  Constant167/1 -> Divide7/1
  [task_time_s] -> Divide7/2
  Constant165/1 -> Switch42/3
  Constant169/1 -> Switch42/2
  Max8/1 -> Switch42/1
  VVMC_ADASACCSta_enum/1 -> [VVMC_ADASACCSta_enum]
  [VVMC_ADASACCSta_enum] -> Relational Operator73/1
  Constant17/1 -> Relational Operator73/2
  Unit Delay1/1 -> Detect Decrease3/1
  Detect Change/1 -> NOT/1
  NOT/1 -> AND/2
  [VVMC_ACCPedalOvrd_flg] -> Unit Delay1/1
  [VVMC_FeatArbitrFinal_enum] -> Unit Delay2/1
  Unit Delay2/1 -> Detect Change/1
  Detect Decrease3/1 -> AND/1
  VVMC_TimeGapJudge_flag/1 -> [VVMC_TimeGapJudge_flag]
  Switch9/1 -> Add5/1
  [VVMC_TimeGapJudge_flag] -> AND31/1
  Constant18/1 -> AND31/2
  AND31/1 -> Switch9/2
  Constant43/1 -> Min3/2
  Constant170/1 -> Switch43/1
  AND32/1 -> Detect Increase8/1
  Constant71/1 -> AND32/3
  Relational Operator27/1 -> AND32/1
  Switch43/1 -> Switch6/3
  [VVMC_ACCDeltaAccel_mps2] -> Relational Operator27/1
  Constant171/1 -> Relational Operator27/2
  Relational Operator74/1 -> AND32/2
  Detect Increase8/1 -> Switch43/2
  Constant172/1 -> Relational Operator74/2
  [VVMC_ActACCRequiredAccel_mps2] -> Relational Operator74/1
  [VVMC_EstSlope_Deg] -> Equal11/1
  Constant173/1 -> Equal11/2
  Equal11/1 -> AND32/4
  Equal12/1 -> AND32/5
  [VVMC_LastADASWhlTqCal_Nm] -> Equal12/1
  Constant174/1 -> Equal12/2
  Saturation Dynamic1/1 -> Switch37/1
  [VVMC_ActACCRequiredAccel_mps2] -> Saturation Dynamic1/2
  Constant139/1 -> Saturation Dynamic1/1
  [VVMC_ActACCRequiredAccel_mps2] -> Switch37/3
  Constant140/1 -> Saturation Dynamic1/3
  Constant138/1 -> Switch37/2
  Switch37/1 -> Add7/1
  Min3/1 -> Switch9/1
  [VVMC_ADASNegReq_flg] -> NOT5/1
  Switch16/1 -> Switch19/3
  NOT5/1 -> Switch16/2
